simulink model "nms_3Dmodel_forward"  (R2017b)
settings: Solver=VariableStepAuto  StartTime=0.0  StopTime=t_end  FixedStep=1e-4  MinStep=1e-9  RelTol=1e-2  AbsTol=1e-3  EnableMultiTasking=on
InitFcn:
  | runScripts;
values from neighbouring files (symbols this model uses):
  ankle_height = 0.08    [nms_MechInit.m]
  ankleIMP = param(91+length(paramIC_opt):93+length(paramIC_opt))    [runScripts.m]
  c = 0.05    [IID_nms_MechInit.m]    (also in nms_MechInit.m)
  c_jointstop = 0.3 / (pi/180)    (= 17.1887338539)    [IID_nms_MechInit.m]    (also in nms_MechInit.m)
  CPG_On = 0    [setCPGPar.m]    (also in setCPGPar_inv.m = 1)
  CtrlPar_FP = [alpha0 alpha_cd alpha_cv]    [setCtrlPar.m]
  CtrlPar_FP_R = [R_hipR0 R_hipR_cd R_hipR_cv]    [setCtrlPar.m]
  CtrlPar_LL = l_clr    [setCtrlPar.m]
  CtrlPar_Side = [beta_cd  beta_cv]    [setCtrlPar.m]
  CtrlPar_St = [StPreStim St_M1 St_M2 St_M3 St_M4 St_M5 St_M11]    [setCtrlPar.m]
  CtrlPar_St_R = [R_StPreStim R_St_M1 R_St_M3 R_St_M4]    [setCtrlPar.m]
  CtrlPar_Sw = [SwPreStim SwPhasePari SwPhaseParii SwCtrlPar_H SwCtrlPar_A      SwCtrlPar_Ki SwCtrlPar_Kii SwCtrlPar_Kiii SwCtrlPar_StP]    [setCtrlPar.m]
  CtrlPar_Sw_R = [R_SwPreStim R_Sw_M6]    [setCtrlPar.m]
  CtrlPar_theta0 = parBlCtrl(1)      *1*pi/180    [setCtrlPar.m]
  CtrlPar_Tr = [Tr_St_sup Tr_Sw]    [setCtrlPar.m]
  CtrlPar_Tr_R = [R_Tr_St_sup R_Tr_Sw]    [setCtrlPar.m]
  D12_F = 0.16    [IID_nms_MechInit.m]    (also in nms_MechInit.m)
  D12_S = L_S    (= 0.5)    [IID_nms_MechInit.m]    (also in nms_MechInit.m = 0.46)
  D12_T = L_T    (= 0.5)    [IID_nms_MechInit.m]    (also in nms_MechInit.m = 0.46)
  D12z_T = 0.1* scalorFactor    (= 0.1)    [nms_MechInit.m]
  D13_F = 0.20    (= 0.2)    [IID_nms_MechInit.m]    (also in nms_MechInit.m)
  D1G_F = 0.14    [IID_nms_MechInit.m]    (also in nms_MechInit.m)
  D1G_HAT = 0.35    [IID_nms_MechInit.m]    (also in nms_MechInit.m)
  D1G_S = 0.3    [IID_nms_MechInit.m]    (also in nms_MechInit.m = 0.28)
  D1G_T = 0.3    [IID_nms_MechInit.m]    (also in nms_MechInit.m = 0.28)
  D1Gy_F = ankle_height*D1G_F/D12_F    (= 0.07)    [nms_MechInit.m]
  d_fBall = 0.1    [nms_MechInit.m]
  d_fHeel = 0.05    [nms_MechInit.m]
  DeltaThRef = 5e-3    (= 0.005)    [IID_nms_MechInit.m]    (also in nms_MechInit.m)
  Dist_LM23_PH = 0    [setDistPar.m]
  Dist_LM34_PH = 0    [setDistPar.m]
  Dist_On = 1    [IID_setDistPar.m]    (also in setDistPar.m)
  Dist_PDur = 0.15    [IID_setDistPar.m]    (also in setDistPar.m)
  Dist_RM23_PH = 0    [setDistPar.m]
  Dist_RM34_PH = 0    [setDistPar.m]
  Dist_StartTime = 15    [IID_setDistPar.m]    (also in setDistPar.m)
  Dist_xyzHAT_front_PH = 0    [setDistPar.m]
  Dist_xyzHAT_sag_PH = 0    [IID_setDistPar.m]    (also in setDistPar.m)
  Dist_xyzLAnkle_PH = 0    [setDistPar.m]
  Dist_xyzRAnkle_PH = 0    [setDistPar.m]
  eref = 0.04    [IID_nms_MechInit.m]    (also in nms_MechInit.m)
  FmaxBFSH = 350    [nms_MechInit.m]
  FmaxGAS = 1500    [IID_nms_MechInit.m]    (also in nms_MechInit.m)
  FmaxGLU = 1500    [IID_nms_MechInit.m]    (also in nms_MechInit.m)
  FmaxHAB = 3000    [nms_MechInit.m]
  FmaxHAD = 4500    [nms_MechInit.m]
  FmaxHAM = 3000    [IID_nms_MechInit.m]    (also in nms_MechInit.m)
  FmaxHFL = 2000    [IID_nms_MechInit.m]    (also in nms_MechInit.m)
  FmaxRF = 1200    [nms_MechInit.m]
  FmaxSOL = 4000    [IID_nms_MechInit.m]    (also in nms_MechInit.m)
  FmaxTA = 800    [IID_nms_MechInit.m]    (also in nms_MechInit.m)
  FmaxVAS = 6000    [IID_nms_MechInit.m]    (also in nms_MechInit.m)
  In_F = 0.005    [IID_nms_MechInit.m]    (also in nms_MechInit.m)
  In_HAT = 3    [IID_nms_MechInit.m]    (also in nms_MechInit.m = 2.5)
  In_S = 0.05    [IID_nms_MechInit.m]    (also in nms_MechInit.m)
  In_T = 0.15    [IID_nms_MechInit.m]    (also in nms_MechInit.m)
  init_a_tgt = 70*pi/180    (= 1.2217304764)    [setInitPar.m]
  init_a_tgtR = 90*pi/180    (= 1.57079632679)    [setInitPar.m]
  Inx_F = 0.0007    [nms_MechInit.m]
  Inx_HAT = 1.0    (= 1)    [nms_MechInit.m]
  Inx_S = 0.003    [nms_MechInit.m]
  Inx_T = 0.03    [nms_MechInit.m]
  Iny_F = 0.005    [nms_MechInit.m]
  Iny_HAT = 4.0    (= 4)    [nms_MechInit.m]
  Iny_S = 0.05    [nms_MechInit.m]
  Iny_T = 0.15    [nms_MechInit.m]
  K = 5    [IID_nms_MechInit.m]    (also in nms_MechInit.m)
  k_gn = k_gn/2    (= 39240)    [nms_MechInit.m]
  k_gt = k_gt/2    (= 3924)    [nms_MechInit.m]
  k_pressure = m_HAT * 9.81 / DeltaThRef    (= 104967)    [IID_nms_MechInit.m]    (also in nms_MechInit.m)
  leg_l = [D12_T D12_S]    [nms_MechInit.m]
  LongDelay = 0.020    (= 0.02)    [IID_setCtrlPar.m]    (also in nms_MechInit.m = 0.01)
  LongLoopDelay = 0.030    (= 0.03)    [nms_MechInit.m]
  loptBFSH = 0.12    [nms_MechInit.m]
  loptGAS = 0.05    [IID_nms_MechInit.m]    (also in nms_MechInit.m)
  loptGLU = 0.11    [IID_nms_MechInit.m]    (also in nms_MechInit.m)
  loptHAB = 0.09    [nms_MechInit.m]
  loptHAD = 0.10    (= 0.1)    [nms_MechInit.m]
  loptHAM = 0.10    (= 0.1)    [IID_nms_MechInit.m]    (also in nms_MechInit.m)
  loptHFL = 0.11    [IID_nms_MechInit.m]    (also in nms_MechInit.m)
  loptRF = 0.08    [nms_MechInit.m]
  loptSOL = 0.04    [IID_nms_MechInit.m]    (also in nms_MechInit.m)
  loptTA = 0.06    [IID_nms_MechInit.m]    (also in nms_MechInit.m)
  loptVAS = 0.08    [IID_nms_MechInit.m]    (also in nms_MechInit.m)
  lslackBFSH = 0.10    (= 0.1)    [nms_MechInit.m]
  lslackGAS = 0.40    (= 0.4)    [IID_nms_MechInit.m]    (also in nms_MechInit.m)
  lslackGLU = 0.13    [IID_nms_MechInit.m]    (also in nms_MechInit.m)
  lslackHAB = 0.07    [nms_MechInit.m]
  lslackHAD = 0.18    [nms_MechInit.m]
  lslackHAM = 0.31    [IID_nms_MechInit.m]    (also in nms_MechInit.m)
  lslackHFL = 0.10    (= 0.1)    [IID_nms_MechInit.m]    (also in nms_MechInit.m)
  lslackRF = 0.35    [nms_MechInit.m]
  lslackSOL = 0.26    [IID_nms_MechInit.m]    (also in nms_MechInit.m)
  lslackTA = 0.24    [IID_nms_MechInit.m]    (also in nms_MechInit.m)
  lslackVAS = 0.23    [IID_nms_MechInit.m]    (also in nms_MechInit.m)
  m_F = 1.25    [IID_nms_MechInit.m]    (also in nms_MechInit.m)
  m_HAT = 53.5    [IID_nms_MechInit.m]    (also in nms_MechInit.m)
  m_S = 3.5    [IID_nms_MechInit.m]    (also in nms_MechInit.m)
  m_T = 8.5    [IID_nms_MechInit.m]    (also in nms_MechInit.m)
  m_Total = m_F*2+m_S*2+m_T*2+m_HAT    (= 80)    [IID_nms_MechInit.m]    (also in nms_MechInit.m)
  massBFSH = 2    [nms_MechInit.m]
  massGAS = 0.45    [IID_nms_MechInit.m]    (also in nms_MechInit.m)
  massGLU = 1.4    [IID_nms_MechInit.m]    (also in nms_MechInit.m)
  massHAB = 1.145    [nms_MechInit.m]
  massHAD = 1.91    [nms_MechInit.m]
  massHAM = 1.82    [IID_nms_MechInit.m]    (also in nms_MechInit.m)
  massHFL = 1.87    [IID_nms_MechInit.m]    (also in nms_MechInit.m)
  massRF = 1    [nms_MechInit.m]
  massSOL = 1.36    [IID_nms_MechInit.m]    (also in nms_MechInit.m)
  massTA = 0.29    [IID_nms_MechInit.m]    (also in nms_MechInit.m)
  massVAS = 2.91    [IID_nms_MechInit.m]    (also in nms_MechInit.m)
  MidDelay = 0.010    (= 0.01)    [IID_setCtrlPar.m]    (also in nms_MechInit.m = 0.005)
  mu_slide = 0.8    [IID_nms_MechInit.m]    (also in nms_MechInit.m)
  mu_stick = 0.9    [IID_nms_MechInit.m]    (also in nms_MechInit.m)
  N = 1.5    [IID_nms_MechInit.m]    (also in cmaes_parfor.m = size(x,1); nms_MechInit.m)
  phi12_LowLimit = 70*pi/180    (= 1.2217304764)    [IID_nms_MechInit.m]    (also in nms_MechInit.m)
  phi12_UpLimit = 130*pi/180    (= 2.26892802759)    [IID_nms_MechInit.m]    (also in nms_MechInit.m)
  phi23_UpLimit = 175*pi/180    (= 3.05432619099)    [IID_nms_MechInit.m]    (also in nms_MechInit.m)
  phi34_UpLimit = 230*pi/180    (= 4.01425727959)    [IID_nms_MechInit.m]    (also in nms_MechInit.m)
  phi34R_LowLimit = -15*pi/180    (= -0.261799387799)    [nms_MechInit.m]
  ... (+115 more)
undefined symbols (not defined in the file or in its folder): Control_type, Fs_prosthesis, magnitude, sgn
libraries: mblibv1 x104, simulink x54, simulink_extras x38, nmc x30, NMCCPG_Library x17, powerlib_meascontrol x5
(part 4 of 17)

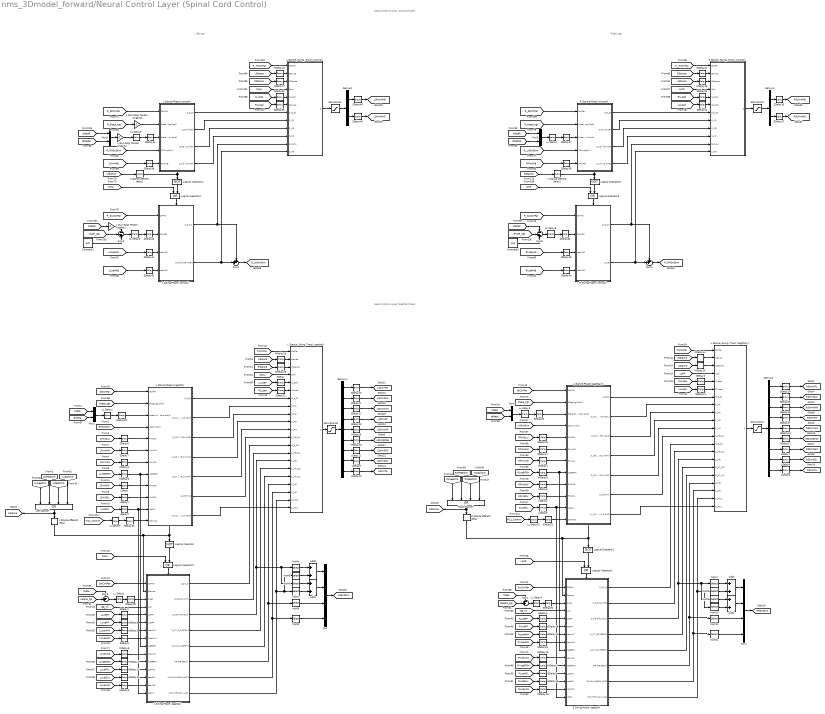
== system nms_3Dmodel_forward/Neural Control Layer (Spinal Cord Control) ==
  note: Neural Control Layer
      | (Sagittal Plane)
  note: Neural Control Layer
      | (Coronal Plane)
  note: Right Leg
  note: Left Leg
  Add{1..3,9} (4 alike) : Sum  Inputs=2
  Constant1 : Constant  Value=pi/2
  Constant2 : Constant  Value=pi/2
  Demux1 : Demux  Outputs=2
  Demux2 : Demux  Outputs=2
  Demux3 : Demux  Outputs=9
  Demux4 : Demux  Outputs=9
  L GLU Golgi Tendon Organs1 : Gain  Gain=-1
  L GLU Golgi Tendon Organs2 : Gain  Gain=-1
  L GLU Golgi Tendon Organs3 : Gain  Gain=-1
  L Stance afferent delay : TransportDelay  DelayTime=MidDelay
  L Stance afferent delay1 : TransportDelay  DelayTime=MidDelay
  L Stance afferent delay2 : TransportDelay  DelayTime=MidDelay
  L Stance Phase (coronal) : Subsystem  TreatAsAtomicUnit=on
  L Stance Phase (sagittal) : Subsystem  TreatAsAtomicUnit=on
  L Stance Phase (sagittal)2 : Subsystem  TreatAsAtomicUnit=on
  "L Stance, Swing, Trans (coronal)" : Subsystem  TreatAsAtomicUnit=on
  "L Stance, Swing, Trans (sagittal)" : Subsystem
  "L Stance, Swing, Trans (sagittal)1" : Subsystem
  L Swing Phase (coronal) : Subsystem  TreatAsAtomicUnit=on
  L Swing Phase (sagittal) : Subsystem  TreatAsAtomicUnit=on
  LDelay{,1,3..4} (4 alike) : TransportDelay  DelayTime=LongDelay
  LDelay10 : TransportDelay  DelayTime=LongDelay  InitialOutput=St_PreSTA
  LDelay11 : TransportDelay  DelayTime=LongDelay  InitialOutput=St_PreSGAS
  LDelay2 : TransportDelay  DelayTime=LongDelay  InitialOutput=1
  LDelay5 : TransportDelay  DelayTime=LongDelay  InitialOutput=1
  LDelay6 : TransportDelay  DelayTime=LongDelay  InitialOutput=Sw_PreSTA
  LDelay7 : TransportDelay  DelayTime=LongDelay  InitialOutput=Sw_PreSGAS
  LDelay8 : TransportDelay  DelayTime=LongDelay  InitialOutput=Sw_PreSSOL
  LDelay9 : TransportDelay  DelayTime=LongDelay  InitialOutput=St_PreSSOL
  LL Delay1 : TransportDelay  DelayTime=LongLoopDelay/2  InitialOutput=init_a_tgt
  LL Delay{2..3,6..7,9..10} (6 alike) : TransportDelay  DelayTime=LongLoopDelay/2
  LL Delay4 : TransportDelay  DelayTime=LongLoopDelay/2  InitialOutput=init_a_tgt
  LL Delay5 : TransportDelay  DelayTime=LongLoopDelay/2  InitialOutput=init_a_tgtR
  LL Delay8 : TransportDelay  DelayTime=LongLoopDelay/2  InitialOutput=init_a_tgtR
  Left Stance? : Logic  Operator=OR  Inputs=4  AllPortsSameDT=off
  Logical Operator{,1,4..5} (4 alike) : Logic  Operator=NOT  AllPortsSameDT=off  OutDataTypeStr=boolean
  Logical Operator{2..3,6..7} (4 alike) : Logic  Operator=OR  AllPortsSameDT=off  OutDataTypeStr=boolean
  MDelay{1..2,4,7..8,13..14,16..22} (14 alike) : TransportDelay  DelayTime=MidDelay
  MDelay10 : TransportDelay  DelayTime=MidDelay  InitialOutput=St_PreSBFSH
  MDelay11 : TransportDelay  DelayTime=MidDelay  InitialOutput=Sw_PreSBFSH
  MDelay12 : TransportDelay  DelayTime=MidDelay  InitialOutput=Sw_PreSVAS
  MDelay{3,5..6,15} (4 alike) : TransportDelay  DelayTime=MidDelay  InitialOutput=1
  MDelay9 : TransportDelay  DelayTime=MidDelay  InitialOutput=St_PreSVAS
  Mux : Mux
  Mux1 : Mux
  Mux{2..5} (4 alike) : Mux  Inputs=2
  R Stance afferent delay : TransportDelay  DelayTime=MidDelay
  R Stance Phase (coronal) : Subsystem  TreatAsAtomicUnit=on
  "R Stance, Swing, Trans (coronal)" : Subsystem  TreatAsAtomicUnit=on
  R Swing Phase (coronal) : Subsystem  TreatAsAtomicUnit=on
  R Swing Phase (sagittal) : Subsystem  TreatAsAtomicUnit=on
  Right Stance? : Logic  Operator=OR  Inputs=4  AllPortsSameDT=off
  SDelay{,3,6..9,12,14,16..19,29..30,32..33,36,38..39,41..42,47,50..51} (24 alike) : TransportDelay  DelayTime=ShortDelay
  SDelay{1..2,4..5,10..11,13,15,34,44..45,49} (12 alike) : TransportDelay  DelayTime=ShortDelay  InitialOutput=1
  SDelay20 : TransportDelay  DelayTime=ShortDelay  InitialOutput=St_PreSHFL
  SDelay21 : TransportDelay  DelayTime=ShortDelay  InitialOutput=St_PreSGLU
  SDelay22 : TransportDelay  DelayTime=ShortDelay  InitialOutput=St_PreSHAM
  SDelay23 : TransportDelay  DelayTime=ShortDelay  InitialOutput=St_PreSRF
  SDelay24 : TransportDelay  DelayTime=ShortDelay  InitialOutput=Sw_PreSHFL
  SDelay25 : TransportDelay  DelayTime=ShortDelay  InitialOutput=Sw_PreSGLU
  SDelay26 : TransportDelay  DelayTime=ShortDelay  InitialOutput=Sw_PreSHAM
  SDelay27 : TransportDelay  DelayTime=ShortDelay  InitialOutput=Sw_PreSRF
  SDelay28 : TransportDelay  DelayTime=ShortDelay  InitialOutput=init_a_tgt
  SDelay31 : TransportDelay  DelayTime=ShortDelay  InitialOutput=init_a_tgt
  SDelay35 : TransportDelay  DelayTime=ShortDelay  InitialOutput=Sw_PreS_HAB
  SDelay37 : TransportDelay  DelayTime=ShortDelay  InitialOutput=Sw_PreS_HAD
  SDelay40 : TransportDelay  DelayTime=ShortDelay  InitialOutput=St_PreS_HAD
  SDelay43 : TransportDelay  DelayTime=ShortDelay  InitialOutput=init_a_tgtR
  SDelay46 : TransportDelay  DelayTime=ShortDelay  InitialOutput=St_PreS_HAB
  SDelay48 : TransportDelay  DelayTime=ShortDelay  InitialOutput=init_a_tgtR
  Saturation{1..3,10} (4 alike) : Saturate  UpperLimit=1  LowerLimit=0.01  ZeroCross=off
  Sum1 : Sum  Inputs=-+|
  Sum2 : Sum  Inputs=++|
  Sum3 : Sum  Inputs=--+
  Sum4 : Sum  Inputs=++|
  Sum5 : Sum  Inputs=--+
  Sum6 : Sum  Inputs=-+|
  hipM{1,4,9,12} (4 alike) : Selector  InputPortWidth=2  IndexOptions=Index vector (dialog)  Indices=1  OutputSizes=1
  hipM10 : Selector  InputPortWidth=3  IndexOptions=Index vector (dialog)  Indices=2  OutputSizes=1
  hipM{2,5,8,11} (4 alike) : Selector  InputPortWidth=3  IndexOptions=Index vector (dialog)  Indices=1  OutputSizes=1
  hipM3 : Selector  InputPortWidth=2  IndexOptions=Index vector (dialog)  Indices=2  OutputSizes=1
  hipM6 : Selector  InputPortWidth=2  IndexOptions=Index vector (dialog)  Indices=2  OutputSizes=1
  hipM7 : Selector  InputPortWidth=3  IndexOptions=Index vector (dialog)  Indices=2  OutputSizes=1
  tag scope: LHSwStim=global, LStance=global, LStimBFSH=global, LStimGAS=global, LStimGLU=global, LStimHAB=global, LStimHAD=global, LStimHAM=global, LStimHFL=global, LStimRF=global, LStimSOL=global, LStimTA=global, LStimVAS=global, RHSwStim=global, RStance=global, RStimBFSH=global, RStimGAS=global, RStimGLU=global, RStimHAB=global, RStimHAD=global, RStimHAM=global, RStimHFL=global, RStimRF=global, RStimSOL=global, RStimTA=global, RStimVAS=global, R_LHSwStim=global, R_RHSwStim=global
  wires:
  [LLLoad] -> SDelay/1
  Left Stance?/1 -> L Stance afferent delay/1, [LStance]
  [StCtrlPar] -> L Stance Phase (sagittal)/1(CtrlPar)
  [RHSwStim] -> L Stance Phase (sagittal)/4(CStim_HSw)
  [LFmGLU] -> SDelay6/1
  SDelay6/1 -> L Stance Phase (sagittal)/5(FmGLU)
  [LFmHAM] -> SDelay7/1
  SDelay7/1 -> L Stance Phase (sagittal)/6(FmHAM)
  [LFmVAS] -> MDelay2/1
  MDelay2/1 -> L Stance Phase (sagittal)/7(FmVAS)
  [LLceBFSH] -> MDelay3/1
  MDelay3/1 -> L Stance Phase (sagittal)/8(LceBFSH), L Swing Phase (sagittal)/9(lceBFSH)
  [LFmGAS] -> LDelay/1
  LDelay/1 -> L Stance Phase (sagittal)/9(FmGAS)
  [LFmSOL] -> LDelay1/1
  LDelay1/1 -> L Stance Phase (sagittal)/10(FmSOL)
  [LLceTA] -> LDelay2/1
  LDelay2/1 -> L Stance Phase (sagittal)/11(LceTA), L Swing Phase (sagittal)/15(LceTA)
  [SwCtrlPar] -> L Swing Phase (sagittal)/1(CtrlPar)
  L Stance afferent delay/1 -> L Stance Phase (sagittal)/Enable, Logical Operator/1, L Swing Phase (sagittal)/2(Stance)
  Logical Operator/1 -> Logical Operator3/2
  Logical Operator3/1 -> L Swing Phase (sagittal)/Enable
  [RonL] -> Logical Operator3/1
  [leg_clr] -> L Swing Phase (sagittal)/4(l_clr)
  [LLceRF] -> SDelay1/1
  SDelay1/1 -> L Swing Phase (sagittal)/5(LceRF)
  [LLceHAM] -> SDelay2/1
  SDelay2/1 -> L Swing Phase (sagittal)/7(LceHAM)
  [LVceRF] -> SDelay8/1
  SDelay8/1 -> L Swing Phase (sagittal)/6(VceRF)
  [LVceHAM] -> SDelay9/1
  SDelay9/1 -> L Swing Phase (sagittal)/8(VceHAM)
  [LVceBFSH] -> MDelay4/1
  MDelay4/1 -> L Swing Phase (sagittal)/11(VceBFSH)
  SDelay10/1 -> L Swing Phase (sagittal)/12(LceHFL)
  SDelay11/1 -> L Swing Phase (sagittal)/13(LceGLU)
  MDelay5/1 -> L Swing Phase (sagittal)/14(LceVAS)
  [TrCtrlPar] -> "L Stance, Swing, Trans (sagittal)"/1(CtrlPar)
  [RLLoad] -> SDelay12/1
  Demux3/1 -> SDelay20/1
  Demux3/2 -> SDelay21/1
  Demux3/3 -> SDelay22/1
  Saturation10/1 -> Demux3/1
  Demux3/7 -> LDelay11/1
  Demux3/8 -> LDelay9/1
  Demux3/9 -> LDelay10/1
  Demux3/4 -> SDelay23/1
  Demux3/5 -> MDelay9/1
  Demux3/6 -> MDelay10/1
  "L Stance, Swing, Trans (sagittal)"/1(S) -> Saturation10/1
  [RonL] -> "L Stance, Swing, Trans (sagittal)"/4(ConI)
  [LStance] -> MDelay20/1
  [RStance] -> MDelay19/1
  Right Stance?/1 -> R Stance afferent delay/1, [RStance]
  [StCtrlPar] -> L Stance Phase (sagittal)2/1(CtrlPar)
  [RLLoad] -> SDelay3/1
  [LHSwStim] -> L Stance Phase (sagittal)2/4(CStim_HSw)
  [RFmGLU] -> SDelay16/1
  SDelay16/1 -> L Stance Phase (sagittal)2/5(FmGLU)
  [RFmHAM] -> SDelay17/1
  SDelay17/1 -> L Stance Phase (sagittal)2/6(FmHAM)
  [RFmVAS] -> MDelay1/1
  MDelay1/1 -> L Stance Phase (sagittal)2/7(FmVAS)
  [RLceBFSH] -> MDelay6/1
  MDelay6/1 -> L Stance Phase (sagittal)2/8(LceBFSH), R Swing Phase (sagittal)/9(lceBFSH)
  [RFmGAS] -> LDelay3/1
  LDelay3/1 -> L Stance Phase (sagittal)2/9(FmGAS)
  [RFmSOL] -> LDelay4/1
  LDelay4/1 -> L Stance Phase (sagittal)2/10(FmSOL)
  [RLceTA] -> LDelay5/1
  LDelay5/1 -> L Stance Phase (sagittal)2/11(LceTA), R Swing Phase (sagittal)/15(LceTA)
  [SwCtrlPar] -> R Swing Phase (sagittal)/1(CtrlPar)
  R Stance afferent delay/1 -> R Swing Phase (sagittal)/2(Stance), L Stance Phase (sagittal)2/Enable, Logical Operator1/1
  Logical Operator1/1 -> Logical Operator2/2
  Logical Operator2/1 -> R Swing Phase (sagittal)/Enable
  [LonR] -> Logical Operator2/1
  [leg_clr] -> R Swing Phase (sagittal)/4(l_clr)
  [RLceRF] -> SDelay4/1
  SDelay4/1 -> R Swing Phase (sagittal)/5(LceRF)
  [RLceHAM] -> SDelay15/1
  SDelay15/1 -> R Swing Phase (sagittal)/7(LceHAM)
  [RVceRF] -> SDelay18/1
  SDelay18/1 -> R Swing Phase (sagittal)/6(VceRF)
  [RVceHAM] -> SDelay19/1
  SDelay19/1 -> R Swing Phase (sagittal)/8(VceHAM)
  [RVceBFSH] -> MDelay7/1
  MDelay7/1 -> R Swing Phase (sagittal)/11(VceBFSH)
  SDelay5/1 -> R Swing Phase (sagittal)/12(LceHFL)
  SDelay13/1 -> R Swing Phase (sagittal)/13(LceGLU)
  MDelay15/1 -> R Swing Phase (sagittal)/14(LceVAS)
  [TrCtrlPar] -> "L Stance, Swing, Trans (sagittal)1"/1(CtrlPar)
  SDelay14/1 -> "L Stance, Swing, Trans (sagittal)1"/6(CLLoad)
  [LLLoad] -> SDelay14/1
  Saturation1/1 -> Demux4/1
  [LonR] -> "L Stance, Swing, Trans (sagittal)1"/4(ConI)
  [RStance] -> MDelay14/1
  [LStance] -> MDelay13/1
  [LLHeelCnt] -> Left Stance?/1
  [LMHeelCnt] -> Left Stance?/2
  [LMBallCnt] -> Left Stance?/3
  [LLBallCnt] -> Left Stance?/4
  [RLHeelCnt] -> Right Stance?/1
  [RMHeelCnt] -> Right Stance?/2
  [RMBallCnt] -> Right Stance?/3
  [RLBallCnt] -> Right Stance?/4
  SDelay12/1 -> "L Stance, Swing, Trans (sagittal)"/6(CLLoad)
  SDelay20/1 -> [LStimHFL]
  SDelay21/1 -> [LStimGLU]
  SDelay22/1 -> [LStimHAM]
  SDelay23/1 -> [LStimRF]
  MDelay9/1 -> [LStimVAS]
  MDelay10/1 -> [LStimBFSH]
  LDelay11/1 -> [LStimGAS]
  LDelay9/1 -> [LStimSOL]
  LDelay10/1 -> [LStimTA]
  Demux4/1 -> SDelay24/1
  Demux4/2 -> SDelay25/1
  Demux4/3 -> SDelay26/1
  Demux4/7 -> LDelay7/1
  Demux4/8 -> LDelay8/1
  Demux4/9 -> LDelay6/1
  Demux4/4 -> SDelay27/1
  Demux4/5 -> MDelay12/1
  Demux4/6 -> MDelay11/1
  SDelay24/1 -> [RStimHFL]
  SDelay25/1 -> [RStimGLU]
  SDelay26/1 -> [RStimHAM]
  SDelay27/1 -> [RStimRF]
  MDelay12/1 -> [RStimVAS]
  MDelay11/1 -> [RStimBFSH]
  LDelay7/1 -> [RStimGAS]
  LDelay8/1 -> [RStimSOL]
  LDelay6/1 -> [RStimTA]
  [Lalpha_tgt] -> Sum6/2
  [theta] -> Sum6/1
  [Ralpha_tgt] -> Sum1/2
  [theta] -> Sum1/1
  MDelay20/1 -> "L Stance, Swing, Trans (sagittal)"/2(Stance)
  MDelay19/1 -> "L Stance, Swing, Trans (sagittal)"/3(CStance)
  MDelay14/1 -> "L Stance, Swing, Trans (sagittal)1"/2(Stance)
  MDelay13/1 -> "L Stance, Swing, Trans (sagittal)1"/3(CStance)
  [LLceHFL] -> SDelay10/1
  [LLceGLU] -> SDelay11/1
  [LLceVAS] -> MDelay5/1
  [RLceHFL] -> SDelay5/1
  [RLceGLU] -> SDelay13/1
  [RLceVAS] -> MDelay15/1
  LL Delay1/1 -> SDelay28/1
  Sum6/1 -> LL Delay1/1
  SDelay28/1 -> L Swing Phase (sagittal)/3(a_tgt)
  L Stance Phase (sagittal)/1(S_St_0) -> "L Stance, Swing, Trans (sagittal)"/7(S_0_St)
  L Swing Phase (sagittal)/1(S_Sw_0) -> "L Stance, Swing, Trans (sagittal)"/13(S_0_Sw)
  L Stance Phase (sagittal)2/1(S_St_0) -> "L Stance, Swing, Trans (sagittal)1"/7(S_0_St)
  L Stance Phase (sagittal)/2(S_M1 [GLU VAS SOL]) -> "L Stance, Swing, Trans (sagittal)"/8(S_M1)
  L Stance Phase (sagittal)/3(S_M2 [HAM VAS BFSH GAS]) -> "L Stance, Swing, Trans (sagittal)"/9(S_M2)
  L Stance Phase (sagittal)/6(S_M5 [TA]) -> "L Stance, Swing, Trans (sagittal)"/12(S_M5_St)
  L Stance Phase (sagittal)2/2(S_M1 [GLU VAS SOL]) -> "L Stance, Swing, Trans (sagittal)1"/8(S_M1)
  L Stance Phase (sagittal)2/3(S_M2 [HAM VAS BFSH GAS]) -> "L Stance, Swing, Trans (sagittal)1"/9(S_M2)
  L Stance Phase (sagittal)2/6(S_M5 [TA]) -> "L Stance, Swing, Trans (sagittal)1"/12(S_M5_St)
  [theta] -> Mux2/1
  [dtheta] -> Mux2/2
  [theta_tgt] -> L Stance Phase (sagittal)/2(theta_tgt [rad])
  SDelay/1 -> "L Stance, Swing, Trans (sagittal)"/5(ILLoad)
  [theta] -> Mux4/1
  [dtheta] -> Mux4/2
  [theta_tgt] -> L Stance Phase (sagittal)2/2(theta_tgt [rad])
  L Stance Phase (sagittal)/4(S_M3 [HFL GLU HAM]) -> "L Stance, Swing, Trans (sagittal)"/10(S_M3)
  L Stance Phase (sagittal)2/4(S_M3 [HFL GLU HAM]) -> "L Stance, Swing, Trans (sagittal)1"/10(S_M3)
  SDelay3/1 -> "L Stance, Swing, Trans (sagittal)1"/5(ILLoad)
  LL Delay2/1 -> SDelay29/1
  Mux2/1 -> LL Delay2/1
  SDelay29/1 -> L Stance Phase (sagittal)/3(theta dtheta [rad rad/s])
  LL Delay3/1 -> SDelay30/1
  Mux4/1 -> LL Delay3/1
  SDelay30/1 -> L Stance Phase (sagittal)2/3(theta dtheta [rad rad/s])
  L Stance Phase (sagittal)2/5(S_M4 [HFL GLU HAM]) -> "L Stance, Swing, Trans (sagittal)1"/11(S_M4)
  L Stance Phase (sagittal)/5(S_M4 [HFL GLU HAM]) -> "L Stance, Swing, Trans (sagittal)"/11(S_M4)
  L Swing Phase (sagittal)/2(S_M5_Sw [TA]) -> "L Stance, Swing, Trans (sagittal)"/14(S_M5_Sw)
  L Swing Phase (sagittal)/3(S_M6 [HFL GLU]) -> "L Stance, Swing, Trans (sagittal)"/15(S_M6), hipM6/1, hipM4/1
  L Swing Phase (sagittal)/4(S_M7_DS [BFSH]) -> "L Stance, Swing, Trans (sagittal)"/16(S_M7_DS)
  L Swing Phase (sagittal)/5(S_M7_Sw [BFSH]) -> "L Stance, Swing, Trans (sagittal)"/17(S_M7_Sw)
  L Swing Phase (sagittal)/6(M8 [RF BFSH]) -> "L Stance, Swing, Trans (sagittal)"/18(S_M8), hipM9/1
  L Swing Phase (sagittal)/7(M9 [HAM BFSH GAS]) -> "L Stance, Swing, Trans (sagittal)"/19(S_M9), hipM8/1
  L Swing Phase (sagittal)/8(M10 [HFL GLU VAS]) -> "L Stance, Swing, Trans (sagittal)"/20(S_M10), hipM5/1, hipM7/1
  Mux/1 -> [LHSwStim]
  hipM4/1 -> Add9/1
  hipM5/1 -> Add9/2
  Add9/1 -> Mux/1
  hipM6/1 -> Add1/1
  hipM7/1 -> Add1/2
  Add1/1 -> Mux/2
  hipM9/1 -> Mux/3
  hipM8/1 -> Mux/4
  "L Stance, Swing, Trans (sagittal)1"/1(S) -> Saturation1/1
  R Swing Phase (sagittal)/1(S_Sw_0) -> "L Stance, Swing, Trans (sagittal)1"/13(S_0_Sw)
  R Swing Phase (sagittal)/2(S_M5_Sw [TA]) -> "L Stance, Swing, Trans (sagittal)1"/14(S_M5_Sw)
  R Swing Phase (sagittal)/3(S_M6 [HFL GLU]) -> "L Stance, Swing, Trans (sagittal)1"/15(S_M6), hipM3/1, hipM1/1
  R Swing Phase (sagittal)/4(S_M7_DS [BFSH]) -> "L Stance, Swing, Trans (sagittal)1"/16(S_M7_DS)
  R Swing Phase (sagittal)/5(S_M7_Sw [BFSH]) -> "L Stance, Swing, Trans (sagittal)1"/17(S_M7_Sw)
  R Swing Phase (sagittal)/6(M8 [RF BFSH]) -> "L Stance, Swing, Trans (sagittal)1"/18(S_M8), hipM12/1
  R Swing Phase (sagittal)/7(M9 [HAM BFSH GAS]) -> "L Stance, Swing, Trans (sagittal)1"/19(S_M9), hipM11/1
  R Swing Phase (sagittal)/8(M10 [HFL GLU VAS]) -> "L Stance, Swing, Trans (sagittal)1"/20(S_M10), hipM2/1, hipM10/1
  Mux1/1 -> [RHSwStim]
  hipM1/1 -> Add3/1
  hipM2/1 -> Add3/2
  Add3/1 -> Mux1/1
  hipM3/1 -> Add2/1
  hipM10/1 -> Add2/2
  Add2/1 -> Mux1/2
  hipM12/1 -> Mux1/3
  hipM11/1 -> Mux1/4
  LL Delay4/1 -> SDelay31/1
  Sum1/1 -> LL Delay4/1
  SDelay31/1 -> R Swing Phase (sagittal)/3(a_tgt)
  [LVceVAS] -> MDelay8/1
  MDelay8/1 -> L Swing Phase (sagittal)/10(VceVAS)
  [RVceVAS] -> MDelay16/1
  MDelay16/1 -> R Swing Phase (sagittal)/10(VceVAS)
  Logical Operator5/1 -> Logical Operator6/2
  Logical Operator6/1 -> R Swing Phase (coronal)/Enable
  [LonR] -> Logical Operator6/1
  [RStance] -> L Stance afferent delay2/1
  L Stance afferent delay2/1 -> Logical Operator5/1, R Stance Phase (coronal)/Enable
  [R_StCtrlPar] -> R Stance Phase (coronal)/1(CtrlPar)
  [R_LHSwStim] -> R Stance Phase (coronal)/4(CSwingStim)
  [R_SwCtrlPar] -> R Swing Phase (coronal)/1(CtrlPar)
  [R_TrCtrlPar] -> "R Stance, Swing, Trans (coronal)"/1(CtrlPar)
  [LonR] -> "R Stance, Swing, Trans (coronal)"/4(ConI)
  [LLLoad] -> SDelay41/1
  SDelay41/1 -> "R Stance, Swing, Trans (coronal)"/6(CLLoad)
  Saturation2/1 -> Demux1/1
  Demux1/2 -> SDelay37/1
  Demux1/1 -> SDelay35/1
  [RLLoad] -> SDelay33/1
  [R_theta_tgt] -> R Stance Phase (coronal)/2(theta_tgt [rad])
  R Swing Phase (coronal)/2(S_M6) -> Sum4/2, "R Stance, Swing, Trans (coronal)"/12(S_M6)
  Sum4/1 -> [R_RHSwStim]
  SDelay33/1 -> "R Stance, Swing, Trans (coronal)"/5(ILLoad)
  R Stance Phase (coronal)/1(S_0_St) -> "R Stance, Swing, Trans (coronal)"/7(S_0_St)
  R Stance Phase (coronal)/3(S_M3 [HAB HAD]) -> "R Stance, Swing, Trans (coronal)"/9(S_M3)
  R Stance Phase (coronal)/4(S_M4 [HAB HAD]) -> "R Stance, Swing, Trans (coronal)"/10(S_M4)
  R Swing Phase (coronal)/1(S_0_Sw) -> Sum4/1, "R Stance, Swing, Trans (coronal)"/11(S_0_Sw)
  [RLceHAD] -> SDelay49/1
  [RLceHAB] -> SDelay34/1
  [RhipR_tgt] -> Sum5/2
  Constant2/1 -> Sum5/3
  [thetaR] -> Sum5/1
  LL Delay7/1 -> SDelay47/1
  SDelay47/1 -> R Stance Phase (coronal)/3(theta dtheta [rad rad/s])
  Mux3/1 -> LL Delay7/1
  LL Delay8/1 -> SDelay48/1
  SDelay48/1 -> R Swing Phase (coronal)/2(R_a_tgt)
  Sum5/1 -> LL Delay8/1
  SDelay49/1 -> R Swing Phase (coronal)/3(LceHAD)
  SDelay34/1 -> R Swing Phase (coronal)/4(LceHAB)
  MDelay21/1 -> "R Stance, Swing, Trans (coronal)"/2(Stance)
  [RStance] -> MDelay21/1
  [LStance] -> MDelay18/1
  MDelay18/1 -> "R Stance, Swing, Trans (coronal)"/3(CStance)
  "R Stance, Swing, Trans (coronal)"/1(S) -> Saturation2/1
  [thetaR] -> Mux3/1
  [dthetaR] -> Mux3/2
  R Stance Phase (coronal)/2(S_M1 [HAB]) -> "R Stance, Swing, Trans (coronal)"/8(S_M1)
  [RFmHAB] -> SDelay38/1
  SDelay38/1 -> R Stance Phase (coronal)/5(FmHAB)
  Logical Operator4/1 -> Logical Operator7/2
  Logical Operator7/1 -> L Swing Phase (coronal)/Enable
  [RonL] -> Logical Operator7/1
  [LStance] -> L Stance afferent delay1/1
  L Stance afferent delay1/1 -> Logical Operator4/1, L Stance Phase (coronal)/Enable
  L GLU Golgi Tendon Organs3/1 -> L Stance Phase (coronal)/2(theta_tgt [rad])
  [R_StCtrlPar] -> L Stance Phase (coronal)/1(CtrlPar)
  [R_RHSwStim] -> L Stance Phase (coronal)/4(CSwingStim)
  [R_SwCtrlPar] -> L Swing Phase (coronal)/1(CtrlPar)
  [R_TrCtrlPar] -> "L Stance, Swing, Trans (coronal)"/1(CtrlPar)
  [RonL] -> "L Stance, Swing, Trans (coronal)"/4(ConI)
  [LStance] -> MDelay22/1
  [RStance] -> MDelay17/1
  [RLLoad] -> SDelay36/1
  SDelay36/1 -> "L Stance, Swing, Trans (coronal)"/6(CLLoad)
  Saturation3/1 -> Demux2/1
  Demux2/2 -> SDelay40/1
  Demux2/1 -> SDelay46/1
  [LLLoad] -> SDelay32/1
  [R_theta_tgt] -> L GLU Golgi Tendon Organs3/1
  Mux5/1 -> L GLU Golgi Tendon Organs1/1
  L Swing Phase (coronal)/2(S_M6 [HAB HAD]) -> Sum2/2, "L Stance, Swing, Trans (coronal)"/12(S_M6)
  Sum2/1 -> [R_LHSwStim]
  SDelay32/1 -> "L Stance, Swing, Trans (coronal)"/5(ILLoad)
  L Stance Phase (coronal)/1(S_0_St) -> "L Stance, Swing, Trans (coronal)"/7(S_0_St)
  L Stance Phase (coronal)/3(S_M3 [HAB HAD]) -> "L Stance, Swing, Trans (coronal)"/9(S_M3)
  L Stance Phase (coronal)/4(S_M4 [HAB HAD]) -> "L Stance, Swing, Trans (coronal)"/10(S_M4)
  L Swing Phase (coronal)/1(S_0_Sw) -> "L Stance, Swing, Trans (coronal)"/11(S_0_Sw), Sum2/1
  [LLceHAD] -> SDelay44/1
  [LLceHAB] -> SDelay45/1
  Constant1/1 -> Sum3/3
  LL Delay6/1 -> SDelay42/1
  SDelay42/1 -> L Stance Phase (coronal)/3(theta dtheta [rad rad/s])
  L GLU Golgi Tendon Organs1/1 -> LL Delay6/1
  LL Delay5/1 -> SDelay43/1
  SDelay43/1 -> L Swing Phase (coronal)/2(R_a_tgt)
  Sum3/1 -> LL Delay5/1
  SDelay44/1 -> L Swing Phase (coronal)/3(LceHAD)
  SDelay45/1 -> L Swing Phase (coronal)/4(LceHAB)
  MDelay22/1 -> "L Stance, Swing, Trans (coronal)"/2(Stance)
  MDelay17/1 -> "L Stance, Swing, Trans (coronal)"/3(CStance)
  SDelay46/1 -> [LStimHAB]
  SDelay40/1 -> [LStimHAD]
  "L Stance, Swing, Trans (coronal)"/1(S) -> Saturation3/1
  [LhipR_tgt] -> Sum3/2
  [thetaR] -> L GLU Golgi Tendon Organs2/1
  L GLU Golgi Tendon Organs2/1 -> Sum3/1
  [thetaR] -> Mux5/1
  [dthetaR] -> Mux5/2
  L Stance Phase (coronal)/2(S_M1 [HAB]) -> "L Stance, Swing, Trans (coronal)"/8(S_M1)
  [LFmHAB] -> SDelay39/1
  SDelay39/1 -> L Stance Phase (coronal)/5(FmHAB)
  SDelay35/1 -> [RStimHAB]
  SDelay37/1 -> [RStimHAD]
  L Stance Phase (sagittal)/7(S_M11 [SOL TA GAS]) -> "L Stance, Swing, Trans (sagittal)"/21(S_M11)
  L Stance Phase (sagittal)2/7(S_M11 [SOL TA GAS]) -> "L Stance, Swing, Trans (sagittal)1"/21(S_M11)
  [M11_Control] -> LL Delay9/1
  [M11_Control] -> LL Delay10/1
  LL Delay9/1 -> SDelay50/1
  SDelay50/1 -> L Stance Phase (sagittal)/12(COMVel)
  LL Delay10/1 -> SDelay51/1
  SDelay51/1 -> L Stance Phase (sagittal)2/12(COMVel)

== system nms_3Dmodel_forward/Positions ==
  Mux : Mux  Inputs=11
  Positions : Outport
  wires:
  Mux/1 -> Positions/1
  [xyzRAnkle] -> Mux/7
  [xyzLKnee] -> Mux/4
  [xyzLHip] -> Mux/5
  [dxyzLHip] -> Mux/6
  [xyzRKnee] -> Mux/8
  [xyzLAnkle] -> Mux/3
  [xyzRHip] -> Mux/9
  [dxyzRHip] -> Mux/10
  [xyzHAT] -> Mux/1
  [dxyzHAT] -> Mux/2
  [xyzTrunk] -> Mux/11

== system nms_3Dmodel_forward/SecondOrderLowPassFilter1 ==
  note: This is an implementation of a
      | second order low pass filter with
      | settable zeta and omega.
      | It works for scalars as well as vectors.
      |
      | You can monitor the output from Python
      | by monitoring OutputValue.s[0,:]
  In : Inport
  Integrator : Integrator
  OutputValue : Integrator  InitialCondition=vx0
  Product1 : Product  RndMeth=Zero
  Product2 : Product  RndMeth=Zero
  Sum : Sum  Inputs=|+-
  Sum1 : Sum  Inputs=|+-
  omega : Constant  Value=w
  omega_sq : Math  Operator=square  SaturateOnIntegerOverflow=on
  two : Constant  Value=2
  zeta : Constant  Value=z
  zeta_omega_2 : Product  Inputs=3  RndMeth=Zero
  Out : Outport
  wires:
  OutputValue/1 -> Out/1, Sum/2
  Sum1/1 -> Integrator/1
  In/1 -> Sum/1
  Integrator/1 -> Product2/1, OutputValue/1
  Sum/1 -> Product1/1
  omega/1 -> zeta_omega_2/3, omega_sq/1
  two/1 -> zeta_omega_2/1
  zeta/1 -> zeta_omega_2/2
  omega_sq/1 -> Product1/2
  Product1/1 -> Sum1/1
  zeta_omega_2/1 -> Product2/2
  Product2/1 -> Sum1/2

== system nms_3Dmodel_forward/Signals NMC Left2 ==
  Mux : Mux  Inputs=11
  signals : Outport
  wires:
  Mux/1 -> signals/1
  [LStimHFL] -> Mux/1
  [LStimGLU] -> Mux/9
  [LStimVAS] -> Mux/3
  [LStimBFSH] -> Mux/7
  [LStimHAD] -> Mux/11
  [LStimSOL] -> Mux/5
  [LStimHAB] -> Mux/10
  [LStimHAM] -> Mux/8
  [LStimGAS] -> Mux/6
  [LStimTA] -> Mux/4
  [LStimRF] -> Mux/2

== system nms_3Dmodel_forward/Signals NMC Left3 ==
  Mux : Mux
  signals : Outport
  wires:
  Mux/1 -> signals/1
  [LM34] -> Mux/1
  [LM23] -> Mux/3
  [LM12] -> Mux/4
  [LM34R] -> Mux/2

== system nms_3Dmodel_forward/Signals NMC Left6 ==
  Mux : Mux  Inputs=11
  signals : Outport
  wires:
  [REnergyRF] -> Mux/2
  [REnergyTA] -> Mux/4
  [REnergyGAS] -> Mux/6
  [REnergyHAM] -> Mux/8
  [REnergyHAB] -> Mux/10
  [REnergySOL] -> Mux/5
  [REnergyHAD] -> Mux/11
  [REnergyBFSH] -> Mux/7
  [REnergyVAS] -> Mux/3
  [REnergyGLU] -> Mux/9
  [REnergyHFL] -> Mux/1
  Mux/1 -> signals/1

== system nms_3Dmodel_forward/Signals NMC Left7 ==
  Mux : Mux  Inputs=11
  signals : Outport
  wires:
  Mux/1 -> signals/1
  [LEnergyHFL] -> Mux/1
  [LEnergyGLU] -> Mux/9
  [LEnergyVAS] -> Mux/3
  [LEnergyBFSH] -> Mux/7
  [LEnergyHAD] -> Mux/11
  [LEnergySOL] -> Mux/5
  [LEnergyHAB] -> Mux/10
  [LEnergyHAM] -> Mux/8
  [LEnergyGAS] -> Mux/6
  [LEnergyTA] -> Mux/4
  [LEnergyRF] -> Mux/2

== system nms_3Dmodel_forward/Signals NMC Right2 ==
  Mux : Mux  Inputs=11
  signals : Outport
  wires:
  [RStimRF] -> Mux/2
  [RStimTA] -> Mux/4
  [RStimGAS] -> Mux/6
  [RStimHAM] -> Mux/8
  [RStimHAB] -> Mux/10
  [RStimSOL] -> Mux/5
  [RStimHAD] -> Mux/11
  [RStimBFSH] -> Mux/7
  [RStimVAS] -> Mux/3
  [RStimGLU] -> Mux/9
  [RStimHFL] -> Mux/1
  Mux/1 -> signals/1

== system nms_3Dmodel_forward/Signals NMC Right3 ==
  Mux : Mux
  signals : Outport
  wires:
  Mux/1 -> signals/1
  [RM34] -> Mux/1
  [RM23] -> Mux/3
  [RM12] -> Mux/4
  [RM34R] -> Mux/2

== system nms_3Dmodel_forward/etc ==
  note: Fall detection
      | (stop simulation)
  note: Control Parameters
  Abs1 : Abs
  Abs3 : Abs
  Clock : Clock
  Compare To Constant2 : simulink/Logic and Bit Operations/Compare To Constant  relop=>  const=60*pi/180  OutDataTypeStr=boolean
  Compare To Constant6 : simulink/Logic and Bit Operations/Compare To Constant  relop=>  const=60*pi/180  OutDataTypeStr=boolean
  Constant1 : Constant  Value=CtrlPar_Side
  Constant10 : Constant  Value=CtrlPar_Tr
  Constant11 : Constant  Value=CtrlPar_Tr_R
  Constant12 : Constant  Value=CtrlPar_theta0
  Constant2 : Constant  Value=CtrlPar_LL
  Constant3 : Constant  Value=CtrlPar_St_R
  Constant5 : Constant  Value=CtrlPar_St
  Constant6 : Constant  Value=CtrlPar_FP
  Constant7 : Constant  Value=CtrlPar_FP_R
  Constant8 : Constant  Value=CtrlPar_Sw_R
  Constant9 : Constant  Value=CtrlPar_Sw
  Logical Operator2 : Logic  Operator=OR  AllPortsSameDT=off  OutDataTypeStr=boolean
  Stop Simulation : Stop
  To Current Workspace2 : ToWorkspace  VariableName=simout_tEnd  SaveFormat=Structure  SampleTime=-1
      settings: MaxDataPoints=1
  tag scope: FPCtrlPar=global, FPCtrlPar_Side=global, LLCtrlPar=global, R_FPCtrlPar=global, R_StCtrlPar=global, R_SwCtrlPar=global, R_TrCtrlPar=global, StCtrlPar=global, SwCtrlPar=global, TrCtrlPar=global, theta0=global
  wires:
  [theta] -> Abs3/1
  Abs3/1 -> Compare To Constant2/1
  Compare To Constant2/1 -> Logical Operator2/1
  Logical Operator2/1 -> Stop Simulation/1
  [thetaR] -> Abs1/1
  Abs1/1 -> Compare To Constant6/1
  Compare To Constant6/1 -> Logical Operator2/2
  Constant6/1 -> [FPCtrlPar]
  Constant9/1 -> [SwCtrlPar]
  Constant2/1 -> [LLCtrlPar]
  Constant5/1 -> [StCtrlPar]
  Constant12/1 -> [theta0]
  Constant3/1 -> [R_StCtrlPar]
  Constant7/1 -> [R_FPCtrlPar]
  Constant8/1 -> [R_SwCtrlPar]
  Constant11/1 -> [R_TrCtrlPar]
  Constant10/1 -> [TrCtrlPar]
  Clock/1 -> To Current Workspace2/1
  Constant1/1 -> [FPCtrlPar_Side]

== system nms_3Dmodel_forward/Body Mechanics Layer/LAnkle ==
  note: 3D Ground Interaction Model
  Dist : Inport
  Body Actuator : mblibv1/Sensors &  Actuators/Body Actuator  UpdateFromCAD=off  PhysicalDomain=Mechanical  PortType=blob  ActuationStyle=Force  AngleUnits=deg  ArcVelocityUnits=deg/s  ArcAccelerationUnits=deg/s^2  CoordPositionUnits=m  VelocityUnits=m/s  AccelerationUnits=m/s^2  ForceUnits=N  TorqueUnits=N*m  ActiveIO=on  Width=3  DialogClass=MechanicalActuatorBlock  ReferenceFrame=Local (Body CS)  Angle=off  CoordPosition=on  Force=on  Torque=off
      settings: SourceProductName=Simscape Multibody  SourceProductBaseCode=MS
  Constant : Constant  Value=0
  Gain : Gain  Gain=-1
  Mechanical Branching Bar : mblibv1/Utilities/Mechanical Branching Bar  LConnTagsString=_newl0  RConnTagsString=SA0|SA1  UpdateFromCAD=off  DialogClass=MechanicalBranchingBarBlock  NumSAPorts=2
      settings: SourceProductName=Simscape Multibody  SourceProductBaseCode=MS
  Mux : Mux  Inputs=3
  Right Heel Sensor15 : mblibv1/Sensors &  Actuators/Body Sensor  UpdateFromCAD=off  PhysicalDomain=Mechanical  PortType=blob  Muxed=off  Pose=off  Angle=on  AngleUnits=deg  ArcVelocity=off  ArcVelocityUnits=deg/s  ArcAcceleration=off  ArcAccelerationUnits=deg/s^2  CoordPosition=on  CoordPositionUnits=m  Velocity=off  VelocityUnits=m/s  Acceleration=off  AccelerationUnits=m/s^2  Quaternion=on  QuaternionDT=off  QuaternionDDT=off  QuaternionUnits=off  OutputVector=[ 3 3 ]  ActiveIO=on  Width=3  DialogClass=MechanicalSensorBlock  ReferenceFrame=Absolute (World)
      settings: SourceProductName=Simscape Multibody  SourceProductBaseCode=MS
  F : PMIOPort  Port=1  Side=Left
  Pos : Outport
  wires:
  Right Heel Sensor15/1 -> Pos/1  "pos"
  Mux/1 -> Body Actuator/1
  Dist/1 -> Gain/1
  Gain/1 -> Mux/2
  Constant/1 -> Mux/3, Mux/1
  connections:
  F/RConn1 -- Mechanical Branching Bar/LConn1
  Mechanical Branching Bar/RConn2 -- Body Actuator/RConn1
  Right Heel Sensor15/LConn1 -- Mechanical Branching Bar/RConn1

== system nms_3Dmodel_forward/Body Mechanics Layer/LLHeelCnt1 ==
  note: 3D Ground Interaction Model
  PosContra : Inport
  3D Contact : Subsystem
  Body Actuator : mblibv1/Sensors &  Actuators/Body Actuator  UpdateFromCAD=off  PhysicalDomain=Mechanical  PortType=blob  ActuationStyle=Force  AngleUnits=deg  ArcVelocityUnits=deg/s  ArcAccelerationUnits=deg/s^2  CoordPositionUnits=m  VelocityUnits=m/s  AccelerationUnits=m/s^2  ForceUnits=N  TorqueUnits=N*m  ActiveIO=on  Width=3  DialogClass=MechanicalActuatorBlock  ReferenceFrame=Absolute (World)  Angle=off  CoordPosition=on  Force=on  Torque=off
      settings: SourceProductName=Simscape Multibody  SourceProductBaseCode=MS
  Body Sensor : mblibv1/Sensors &  Actuators/Body Sensor  UpdateFromCAD=off  PhysicalDomain=Mechanical  PortType=blob  Muxed=off  Pose=off  Angle=on  AngleUnits=deg  ArcVelocity=off  ArcVelocityUnits=deg/s  ArcAcceleration=off  ArcAccelerationUnits=deg/s^2  CoordPosition=on  CoordPositionUnits=m  Velocity=on  VelocityUnits=m/s  Acceleration=off  AccelerationUnits=m/s^2  Quaternion=on  QuaternionDT=off  QuaternionDDT=off  QuaternionUnits=off  OutputVector=[ 3 3 ]  ActiveIO=on  Width=6  DialogClass=MechanicalSensorBlock  ReferenceFrame=Absolute (World)
      settings: SourceProductName=Simscape Multibody  SourceProductBaseCode=MS
  Demux1 : Demux  Outputs=3
  GroundFunction : nmc/GroundFunction
      settings: SourceProductName=Neuro Muscular Controller Library
  Mechanical Branching Bar : mblibv1/Utilities/Mechanical Branching Bar  LConnTagsString=_newl0  RConnTagsString=SA0|SA1  UpdateFromCAD=off  DialogClass=MechanicalBranchingBarBlock  NumSAPorts=2
      settings: SourceProductName=Simscape Multibody  SourceProductBaseCode=MS
  Mux : Mux  Inputs=3
  Sum : Sum  Inputs=|+-
  Sum1 : Sum
  Terminator : Terminator
  contact? : simulink/Logic and Bit Operations/Compare To Zero  relop=<=  OutDataTypeStr=boolean
  y : Selector  InputPortWidth=3  IndexOptions=Index vector (dialog)  Indices=2  OutputSizes=1
  F : PMIOPort  Port=1  Side=Left
  RBallCnt : Outport
  tag scope: LMHeelF=global
  wires:
  GroundFunction/2 -> 3D Contact/2(nVec [m m m])
  GroundFunction/1 -> Mux/2, Sum/2
  Demux1/2 -> Terminator/1
  Demux1/3 -> Mux/3
  Demux1/1 -> Mux/1
  Mux/1 -> 3D Contact/1(RefPt [m m m])  "Reference Point RefPt"
  y/1 -> Sum/1
  Sum/1 -> contact?/1
  3D Contact/2(FtVec [N N N]) -> Sum1/2
  3D Contact/1(FnVec [N N N]) -> Sum1/1
  Body Sensor/2 -> 3D Contact/4(vVec [m/s m/s m/s])
  Body Sensor/1 -> y/1, Demux1/1, 3D Contact/3(pVec [m m m])  "pos"
  contact?/1 -> RBallCnt/1, 3D Contact/Enable  "cnt"
  PosContra/1 -> GroundFunction/1
  Sum1/1 -> [LMHeelF], Body Actuator/1
  connections:
  Mechanical Branching Bar/RConn1 -- Body Sensor/LConn1
  Mechanical Branching Bar/RConn2 -- Body Actuator/RConn1
  F/RConn1 -- Mechanical Branching Bar/LConn1

== system nms_3Dmodel_forward/Body Mechanics Layer/LLHeelCnt2 ==
  note: 3D Ground Interaction Model
  PosContra : Inport
  3D Contact : Subsystem
  Body Actuator : mblibv1/Sensors &  Actuators/Body Actuator  UpdateFromCAD=off  PhysicalDomain=Mechanical  PortType=blob  ActuationStyle=Force  AngleUnits=deg  ArcVelocityUnits=deg/s  ArcAccelerationUnits=deg/s^2  CoordPositionUnits=m  VelocityUnits=m/s  AccelerationUnits=m/s^2  ForceUnits=N  TorqueUnits=N*m  ActiveIO=on  Width=3  DialogClass=MechanicalActuatorBlock  ReferenceFrame=Absolute (World)  Angle=off  CoordPosition=on  Force=on  Torque=off
      settings: SourceProductName=Simscape Multibody  SourceProductBaseCode=MS
  Body Sensor : mblibv1/Sensors &  Actuators/Body Sensor  UpdateFromCAD=off  PhysicalDomain=Mechanical  PortType=blob  Muxed=off  Pose=off  Angle=on  AngleUnits=deg  ArcVelocity=off  ArcVelocityUnits=deg/s  ArcAcceleration=off  ArcAccelerationUnits=deg/s^2  CoordPosition=on  CoordPositionUnits=m  Velocity=on  VelocityUnits=m/s  Acceleration=off  AccelerationUnits=m/s^2  Quaternion=on  QuaternionDT=off  QuaternionDDT=off  QuaternionUnits=off  OutputVector=[ 3 3 ]  ActiveIO=on  Width=6  DialogClass=MechanicalSensorBlock  ReferenceFrame=Absolute (World)
      settings: SourceProductName=Simscape Multibody  SourceProductBaseCode=MS
  Demux1 : Demux  Outputs=3
  GroundFunction : nmc/GroundFunction
      settings: SourceProductName=Neuro Muscular Controller Library
  Mechanical Branching Bar : mblibv1/Utilities/Mechanical Branching Bar  LConnTagsString=_newl0  RConnTagsString=SA0|SA1  UpdateFromCAD=off  DialogClass=MechanicalBranchingBarBlock  NumSAPorts=2
      settings: SourceProductName=Simscape Multibody  SourceProductBaseCode=MS
  Mux : Mux  Inputs=3
  Sum : Sum  Inputs=|+-
  Sum1 : Sum
  Terminator : Terminator
  contact? : simulink/Logic and Bit Operations/Compare To Zero  relop=<=  OutDataTypeStr=boolean
  y : Selector  InputPortWidth=3  IndexOptions=Index vector (dialog)  Indices=2  OutputSizes=1
  F : PMIOPort  Port=1  Side=Left
  RBallCnt : Outport
  tag scope: LLBallF=global
  wires:
  GroundFunction/2 -> 3D Contact/2(nVec [m m m])
  GroundFunction/1 -> Mux/2, Sum/2
  Demux1/2 -> Terminator/1
  Demux1/3 -> Mux/3
  Demux1/1 -> Mux/1
  Mux/1 -> 3D Contact/1(RefPt [m m m])  "Reference Point RefPt"
  y/1 -> Sum/1
  Sum/1 -> contact?/1
  3D Contact/2(FtVec [N N N]) -> Sum1/2
  3D Contact/1(FnVec [N N N]) -> Sum1/1
  Body Sensor/2 -> 3D Contact/4(vVec [m/s m/s m/s])
  Body Sensor/1 -> y/1, Demux1/1, 3D Contact/3(pVec [m m m])  "pos"
  contact?/1 -> RBallCnt/1, 3D Contact/Enable  "cnt"
  PosContra/1 -> GroundFunction/1
  Sum1/1 -> [LLBallF], Body Actuator/1
  connections:
  Mechanical Branching Bar/RConn1 -- Body Sensor/LConn1
  Mechanical Branching Bar/RConn2 -- Body Actuator/RConn1
  F/RConn1 -- Mechanical Branching Bar/LConn1

== system nms_3Dmodel_forward/Body Mechanics Layer/LLHeelCnt3 ==
  note: 3D Ground Interaction Model
  3D Contact : Subsystem
  Body Actuator : mblibv1/Sensors &  Actuators/Body Actuator  UpdateFromCAD=off  PhysicalDomain=Mechanical  PortType=blob  ActuationStyle=Force  AngleUnits=deg  ArcVelocityUnits=deg/s  ArcAccelerationUnits=deg/s^2  CoordPositionUnits=m  VelocityUnits=m/s  AccelerationUnits=m/s^2  ForceUnits=N  TorqueUnits=N*m  ActiveIO=on  Width=3  DialogClass=MechanicalActuatorBlock  ReferenceFrame=Absolute (World)  Angle=off  CoordPosition=on  Force=on  Torque=off
      settings: SourceProductName=Simscape Multibody  SourceProductBaseCode=MS
  Body Sensor : mblibv1/Sensors &  Actuators/Body Sensor  UpdateFromCAD=off  PhysicalDomain=Mechanical  PortType=blob  Muxed=off  Pose=off  Angle=on  AngleUnits=deg  ArcVelocity=off  ArcVelocityUnits=deg/s  ArcAcceleration=off  ArcAccelerationUnits=deg/s^2  CoordPosition=on  CoordPositionUnits=m  Velocity=on  VelocityUnits=m/s  Acceleration=off  AccelerationUnits=m/s^2  Quaternion=on  QuaternionDT=off  QuaternionDDT=off  QuaternionUnits=off  OutputVector=[ 3 3 ]  ActiveIO=on  Width=6  DialogClass=MechanicalSensorBlock  ReferenceFrame=Absolute (World)
      settings: SourceProductName=Simscape Multibody  SourceProductBaseCode=MS
  Demux1 : Demux  Outputs=3
  GroundFunction : nmc/GroundFunction
      settings: SourceProductName=Neuro Muscular Controller Library
  Mechanical Branching Bar : mblibv1/Utilities/Mechanical Branching Bar  LConnTagsString=_newl0  RConnTagsString=SA0|SA1  UpdateFromCAD=off  DialogClass=MechanicalBranchingBarBlock  NumSAPorts=2
      settings: SourceProductName=Simscape Multibody  SourceProductBaseCode=MS
  Mux : Mux  Inputs=3
  Sum : Sum  Inputs=|+-
  Sum1 : Sum
  Terminator : Terminator
  contact? : simulink/Logic and Bit Operations/Compare To Zero  relop=<=  OutDataTypeStr=boolean
  y : Selector  InputPortWidth=3  IndexOptions=Index vector (dialog)  Indices=2  OutputSizes=1
  F : PMIOPort  Port=1  Side=Left
  RBallCnt : Outport
  RBallCnt1 : Outport  Port=2
  tag scope: LMBallF=global
  wires:
  contact?/1 -> 3D Contact/Enable, RBallCnt/1  "cnt"
  Body Sensor/1 -> RBallCnt1/1, GroundFunction/1, 3D Contact/3(pVec [m m m]), Demux1/1, y/1  "pos"
  Body Sensor/2 -> 3D Contact/4(vVec [m/s m/s m/s])
  3D Contact/1(FnVec [N N N]) -> Sum1/1
  3D Contact/2(FtVec [N N N]) -> Sum1/2
  Sum/1 -> contact?/1
  y/1 -> Sum/1
  Mux/1 -> 3D Contact/1(RefPt [m m m])  "Reference Point RefPt"
  Demux1/1 -> Mux/1
  Demux1/3 -> Mux/3
  Demux1/2 -> Terminator/1
  GroundFunction/1 -> Sum/2, Mux/2
  GroundFunction/2 -> 3D Contact/2(nVec [m m m])
  Sum1/1 -> [LMBallF], Body Actuator/1
  connections:
  F/RConn1 -- Mechanical Branching Bar/LConn1
  Mechanical Branching Bar/RConn2 -- Body Actuator/RConn1
  Mechanical Branching Bar/RConn1 -- Body Sensor/LConn1

== system nms_3Dmodel_forward/Body Mechanics Layer/LLHeelCnt4 ==
  note: 3D Ground Interaction Model
  3D Contact : Subsystem
  Body Actuator : mblibv1/Sensors &  Actuators/Body Actuator  UpdateFromCAD=off  PhysicalDomain=Mechanical  PortType=blob  ActuationStyle=Force  AngleUnits=deg  ArcVelocityUnits=deg/s  ArcAccelerationUnits=deg/s^2  CoordPositionUnits=m  VelocityUnits=m/s  AccelerationUnits=m/s^2  ForceUnits=N  TorqueUnits=N*m  ActiveIO=on  Width=3  DialogClass=MechanicalActuatorBlock  ReferenceFrame=Absolute (World)  Angle=off  CoordPosition=on  Force=on  Torque=off
      settings: SourceProductName=Simscape Multibody  SourceProductBaseCode=MS
  Body Sensor : mblibv1/Sensors &  Actuators/Body Sensor  UpdateFromCAD=off  PhysicalDomain=Mechanical  PortType=blob  Muxed=off  Pose=off  Angle=on  AngleUnits=deg  ArcVelocity=off  ArcVelocityUnits=deg/s  ArcAcceleration=off  ArcAccelerationUnits=deg/s^2  CoordPosition=on  CoordPositionUnits=m  Velocity=on  VelocityUnits=m/s  Acceleration=off  AccelerationUnits=m/s^2  Quaternion=on  QuaternionDT=off  QuaternionDDT=off  QuaternionUnits=off  OutputVector=[ 3 3 ]  ActiveIO=on  Width=6  DialogClass=MechanicalSensorBlock  ReferenceFrame=Absolute (World)
      settings: SourceProductName=Simscape Multibody  SourceProductBaseCode=MS
  Demux1 : Demux  Outputs=3
  GroundFunction : nmc/GroundFunction
      settings: SourceProductName=Neuro Muscular Controller Library
  Mechanical Branching Bar : mblibv1/Utilities/Mechanical Branching Bar  LConnTagsString=_newl0  RConnTagsString=SA0|SA1  UpdateFromCAD=off  DialogClass=MechanicalBranchingBarBlock  NumSAPorts=2
      settings: SourceProductName=Simscape Multibody  SourceProductBaseCode=MS
  Mux : Mux  Inputs=3
  Scope : Scope
  Scope1 : Scope
  Sum : Sum  Inputs=|+-
  Sum1 : Sum
  Terminator : Terminator
  contact? : simulink/Logic and Bit Operations/Compare To Zero  relop=<=  OutDataTypeStr=boolean
  y : Selector  InputPortWidth=3  IndexOptions=Index vector (dialog)  Indices=2  OutputSizes=1
  F : PMIOPort  Port=1  Side=Left
  RBallCnt : Outport
  RBallCnt1 : Outport  Port=2
  tag scope: LLHeelF=global
  wires:
  contact?/1 -> 3D Contact/Enable, RBallCnt/1  "cnt"
  Body Sensor/1 -> RBallCnt1/1, GroundFunction/1, 3D Contact/3(pVec [m m m]), Demux1/1, y/1  "pos"
  Body Sensor/2 -> 3D Contact/4(vVec [m/s m/s m/s])
  3D Contact/1(FnVec [N N N]) -> Sum1/1
  3D Contact/2(FtVec [N N N]) -> Sum1/2
  Sum/1 -> contact?/1
  y/1 -> Sum/1
  Mux/1 -> 3D Contact/1(RefPt [m m m])  "Reference Point RefPt"
  Demux1/1 -> Mux/1
  Demux1/3 -> Mux/3
  Demux1/2 -> Terminator/1
  GroundFunction/1 -> Sum/2, Mux/2, Scope/1
  Sum1/1 -> [LLHeelF], Body Actuator/1
  GroundFunction/2 -> Scope1/1, 3D Contact/2(nVec [m m m])
  connections:
  F/RConn1 -- Mechanical Branching Bar/LConn1
  Mechanical Branching Bar/RConn2 -- Body Actuator/RConn1
  Mechanical Branching Bar/RConn1 -- Body Sensor/LConn1
